simulink model "pid_dt_example"  (Simulink 7.6)
settings: Solver=ode45  StartTime=0.0  StopTime=10.0  RelTol=1e-3
settings Model: Creator=nkottens  LastModifiedBy=nkottens

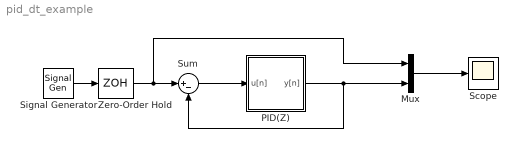
== system pid_dt_example ==
  Mux : Mux  Inputs=2
  PID(Z) : Subsystem  mask{Kp=1, Ki=1, Kd=1, tau=.01/pi, Ts=.01}
      mask prompts: Ts "sampling time (seconds)"
      mask init:
      | Hs=tf([Kp*tau+Kd,Ki*tau+Kp,Ki],[tau,1,0]);
      | Hz=c2d(Hs,Ts,'tustin');
      | %figure(1);bode(Hs,Hz);grid;
      | %figure(2);nyquist(Hs,Hz);grid;
  Scope : Scope
  Signal Generator : SignalGenerator
  Sum : Sum  Inputs=|+-
  Zero-Order Hold : ZeroOrderHold  SampleTime=.01
  wires:
  Sum/1 -> PID(Z)/1(u[n])
  PID(Z)/1(y[n]) -> Sum/2, Mux/2
  Signal Generator/1 -> Zero-Order Hold/1
  Mux/1 -> Scope/1
  Zero-Order Hold/1 -> Sum/1, Mux/1

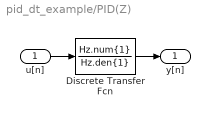
== system pid_dt_example/PID(Z) ==
  u[n] : Inport
  Discrete Transfer Fcn : DiscreteTransferFcn  Numerator=Hz.num{1}  Denominator=Hz.den{1}  SampleTime=Ts
  y[n] : Outport
  wires:
  u[n]/1 -> Discrete Transfer Fcn/1
  Discrete Transfer Fcn/1 -> y[n]/1
